simulink model "PRBS_Pattern_Detector"  (R2021a)
settings: Solver=VariableStepAuto  StartTime=0.0  StopTime=10.0  RelTol=1e-3
libraries: msbAdcFoundation x1
settings Model: Creator=MGMA  LastModifiedBy=MGMA

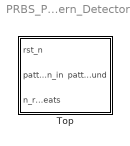
== system PRBS_Pattern_Detector ==
  Top : Subsystem

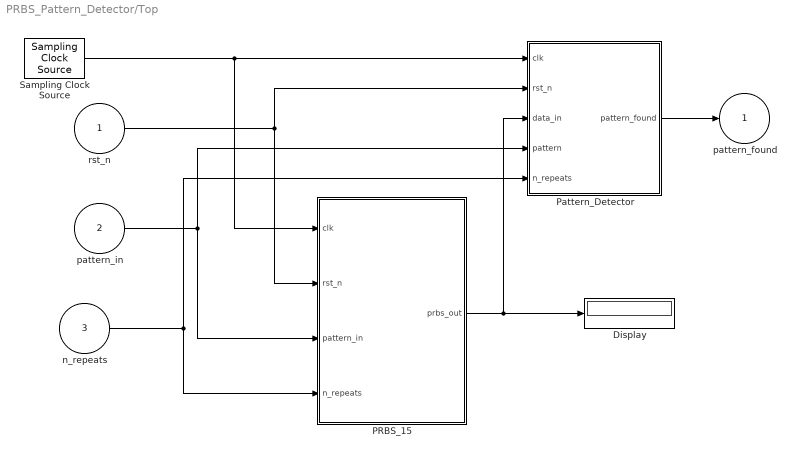
== system PRBS_Pattern_Detector/Top ==
  rst_n : Inport
  pattern_in : Inport  Port=2
  n_repeats : Inport  Port=3
  Display : Display
  PRBS_15 : Subsystem
  Pattern_Detector : Subsystem
  Sampling Clock Source : msbAdcFoundation/Sampling Clock Source  Freq=1e6  Min=0  Max=1  RmsJitt=1e-12  ExtraBuffer=off  NBuffer=50
      settings: SourceProductBaseCode=AM  SignalType=Square wave
  pattern_found : Outport
  wires:
  rst_n/1 -> Pattern_Detector/2(rst_n), PRBS_15/2(rst_n)
  pattern_in/1 -> PRBS_15/3(pattern_in), Pattern_Detector/4(pattern)
  n_repeats/1 -> Pattern_Detector/5(n_repeats), PRBS_15/4(n_repeats)
  PRBS_15/1(prbs_out) -> Display/1, Pattern_Detector/3(data_in)
  Sampling Clock Source/1 -> Pattern_Detector/1(clk), PRBS_15/1(clk)
  Pattern_Detector/1(pattern_found) -> pattern_found/1

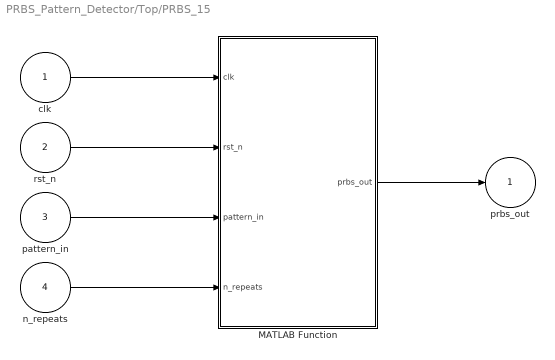
== system PRBS_Pattern_Detector/Top/PRBS_15 ==
  clk : Inport
  rst_n : Inport  Port=2
  pattern_in : Inport  Port=3
  n_repeats : Inport  Port=4
  MATLAB Function : MATLAB Function  TreatAsAtomicUnit=on
  prbs_out : Outport
  wires:
  MATLAB Function/1(prbs_out) -> prbs_out/1
  clk/1 -> MATLAB Function/1(clk)
  rst_n/1 -> MATLAB Function/2(rst_n)
  n_repeats/1 -> MATLAB Function/4(n_repeats)
  pattern_in/1 -> MATLAB Function/3(pattern_in)

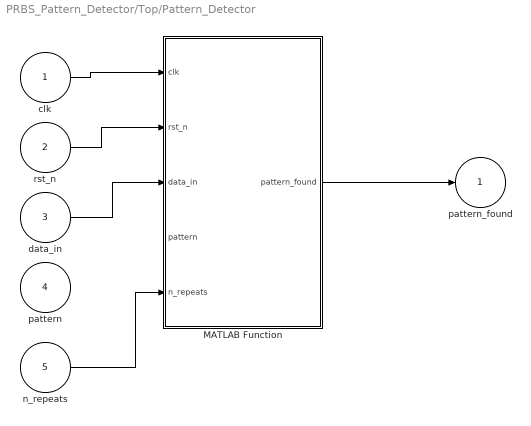
== system PRBS_Pattern_Detector/Top/Pattern_Detector ==
  clk : Inport
  rst_n : Inport  Port=2
  data_in : Inport  Port=3
  pattern : Inport  Port=4
  n_repeats : Inport  Port=5
  MATLAB Function : MATLAB Function  TreatAsAtomicUnit=on
  pattern_found : Outport
  wires:
  MATLAB Function/1(pattern_found) -> pattern_found/1
  clk/1 -> MATLAB Function/1(clk)
  rst_n/1 -> MATLAB Function/2(rst_n)
  data_in/1 -> MATLAB Function/3(data_in)
  n_repeats/1 -> MATLAB Function/5(n_repeats)

== matlab function PRBS_Pattern_Detector/Top/PRBS_15/MATLAB Function ==
  data: clk input; prbs_out output; rst_n input; pattern_in input; n_repeats input
function prbs_out = PRBS_15(clk, rst_n, pattern_in, n_repeats)
    % Initialize variables
    persistent pattern_counter byte_counter prbs_out_reg;
    
    if isempty(pattern_counter)
        pattern_counter = 0;
        byte_counter = 0;
        prbs_out_reg = uint8(255);  % 8'hFF in Verilog
    end
    
    % Reset condition
    if rst_n == 0 || n_repeats == 0
        prbs_out_reg = uint8(255);  % Reset the output to 8'hFF
        pattern_counter = 0;
        prbs_out_reg = 0;
        byte_counter = 0;
    else
        % PRBS generation logic
        if pattern_counter < n_repeats
            % Determine the current byte based on the byte_counter
            switch byte_counter
                case 0
                    prbs_out_reg = bitshift(pattern_in, -24); % pattern_in[31:24]
                case 1
                    prbs_out_reg = bitshift(bitand(pattern_in, 16711680), -16); % pattern_in[23:16]
                case 2
                    prbs_out_reg = bitshift(bitand(pattern_in, 65280), -8); % pattern_in[15:8]
                case 3
                    prbs_out_reg = bitand(pattern_in, 255); % pattern_in[7:0]
                otherwise
                    prbs_out_reg = uint8(255);  % Default case
            end

            % Update the byte counter
            if byte_counter < 3
                byte_counter = byte_counter + 1;
            else
                byte_counter = 0;
                pattern_counter = pattern_counter + 1;
            end
        else
            % Shift and XOR logic for the PRBS sequence
            if byte_counter < 3
                prbs_out_reg = bitshift(prbs_out_reg, -1);
                prbs_out_reg = bitor(prbs_out_reg, bitshift(bitxor(bitget(pattern_in, 14), bitget(pattern_in, 15)), 7));
                byte_counter = byte_counter + 1;
            else
                byte_counter = 0;
                pattern_counter = 0;
            end
        end
    end

    % Output the result
    prbs_out = prbs_out_reg;
end

== matlab function PRBS_Pattern_Detector/Top/Pattern_Detector/MATLAB Function ==
  data: clk input; pattern_found output; rst_n input; data_in input; pattern input; n_repeats input
function pattern_found = Pattern_Detector(clk, rst_n, data_in, pattern, n_repeats)
    % Initialize persistent variables to store states between clock cycles
    persistent current_state next_state pattern_counter byte_counter;
    persistent pattern_found_reg;

    % Define the state values for the FSM
    IDLE = uint8(0);
    MATCHING = uint8(1);
    FOUND = uint8(2);

    if isempty(current_state)
        current_state = IDLE;
        next_state = IDLE;
        pattern_counter = 0;
        byte_counter = 0;
        pattern_found_reg = 0;
    end

    % Handle the reset condition
    if rst_n == 0
        current_state = IDLE;
        next_state = IDLE;
        pattern_counter = 0;
        byte_counter = 0;
        pattern_found_reg = 0;
    else
        % State transition logic
        current_state = next_state;

        % State machine logic
        switch current_state
            case IDLE
                if data_in == bitshift(pattern, -24)  % pattern[31:24]
                    pattern_counter = 1;
                    byte_counter = 1;
                    next_state = MATCHING;
                else
                    pattern_counter = 0;
                    byte_counter = 0;
                    next_state = IDLE;
                end

            case MATCHING
                switch byte_counter
                    case 0
                        if data_in == bitshift(pattern, -24)  % pattern[31:24]
                            byte_counter = byte_counter + 1;
                        end
                    case 1
                        if data_in == bitshift(bitand(pattern, 16711680), -16)  % pattern[23:16]
                            byte_counter = byte_counter + 1;
                        end
                    case 2
                        if data_in == bitshift(bitand(pattern, 65280), -8)  % pattern[15:8]
                            byte_counter = byte_counter + 1;
                        end
                    case 3
                        if data_in == bitand(pattern, 255)  % pattern[7:0]
                            byte_counter = 0;
                            pattern_counter = pattern_counter + 1;

                            if pattern_counter > n_repeats
                                pattern_found_reg = 1;
                                next_state = FOUND;
                            end
                        else
                            pattern_counter = 0;
                            next_state = IDLE;
                        end
                end

            case FOUND
                pattern_found_reg = 1;

            otherwise
                next_state = IDLE;
        end
    end

    % Output the result
    pattern_found = pattern_found_reg;
end
